simulink model "TestaBlocosUteis2"  (R2020b)
settings: Solver=FixedStepDiscrete  StartTime=0.0  StopTime=Plano.Tempo(end)  FixedStep=1  RelTol=1e-3
InitFcn:
  | CarregaTabelas
  | Plano=readtable('PlanoExperimentos.xlsx');
  | FreqIni=Plano.Frequencia(1);
  | PChegadaIni=Plano.PMonAlvo(1);
  | PSucIni=Interpola(FreqIni,PChegadaIni,TabSimulador,8);
  | VazaoIni=Interpola(FreqIni,PChegadaIni,TabSimulador,3);
  | FreqAlvoIni=FreqIni+1;
  | PMonAlvoIni=PChegadaIni+1;
  | VazaoAlvoIni=Interpola(FreqAlvoIni,PMonAlvoIni*1.019716,TabSimulador,3);
values from neighbouring files (symbols this model uses):
  BTP = readtable('DoBTP.xlsx')    [CarregaTabelas.m]
  TabSimulador = LeConverteNomes('DoSimulador.xlsx')    [CarregaTabelas.m]
undefined symbols (not defined in the file or in its folder): Interpola
settings Model: Creator=leize  LastModifiedBy=leize

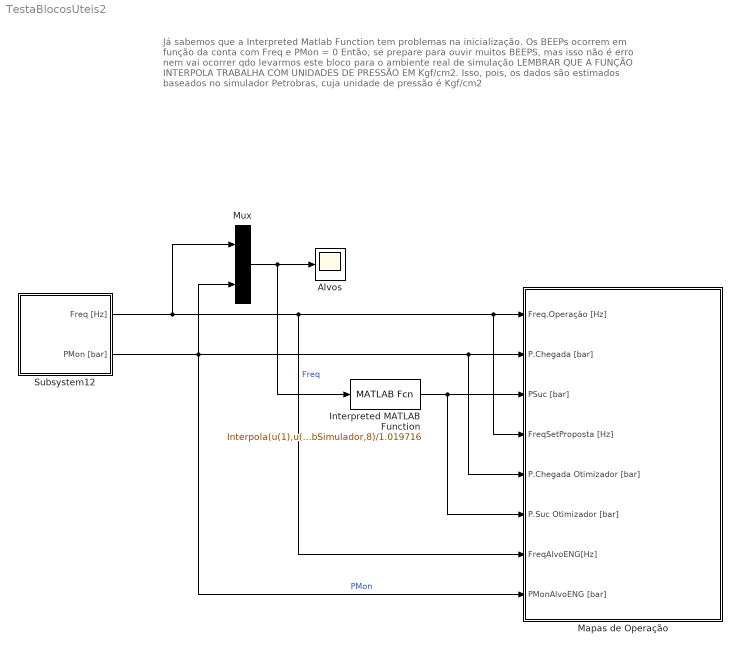
== system TestaBlocosUteis2 ==
  note: Já sabemos que a Interpreted Matlab Function tem problemas na inicialização.
      |
      | Os BEEPs ocorrem em função da conta com Freq e PMon = 0
      |
      | Então, se prepare para ouvir muitos BEEPS, mas isso não é erro nem vai ocorrer qdo levarmos este bloco para o ambiente real de simulação
      |
      | LEMBRAR QUE A FUNÇÃO INTERPOLA TRABALHA COM UNIDADES DE PRESSÃO EM Kgf/cm2. Isso, pois, os dados são estimados baseados no simulador Petrobras, cuja unidade de pressão é Kgf/cm2
  Alvos : Scope
  Interpreted MATLAB Function : MATLABFcn  MATLABFcn=Interpola(u(1),u(2)*1.019716,TabSimulador,8)/1.019716
  Mapas de Operação : Subsystem  mask{PlotaMapas=1, HabilitaRastro=1, Tsim=TabSimulador, BTP=BTP, FreqIni=FreqIni, PChegadaIni=PChegadaIni, PSucIni=PSucIni, FreqAlvoIni=FreqAlvoIni, PMonAlvoIni=PMonAlvoIni}
      mask prompts: PlotaMapas "Plotar Mapas (1/0)?"; HabilitaRastro "Habilita Rastro do Plot (1/0)?"; Tsim "Tabela do Simulador"; BTP "Tabela BTP"; FreqIni "Frequencia Inicial [Hz]"; PChegadaIni "PChegada Inicial [bar]"; PSucIni "Pressao de Succao Inicial [bar]"; FreqAlvoIni "Frequencia ALVO Inicial [Hz]"; PMonAlvoIni "PChegada ALVO [bar]"
      mask DialogControl DescTextVar Prompt: MAPAS DE OPERAÇÃO
      mask DialogControl ParameterGroupVar Prompt: Tabelas Petrobras e configurações dos Mapas de Operação
      mask DialogControl ParameterGroupVar_copy Prompt: Dados do Processo
      mask DialogControl ParameterGroupVar_copy_copy_copy Prompt: Dados Engenharia (Alvos)
  Mux : Mux  Inputs=2
  Subsystem12 : Subsystem  mask{Plano=Plano}
      mask prompts: Plano "Plano de Execucao"
      mask DialogControl DescGroupVar Prompt: TABELA COM PLANO DE EXECUCAO
  wires:
  Mux/1 -> Alvos/1, Interpreted MATLAB Function/1
  Subsystem12/2(PMon [bar]) -> Mapas de Operação/8(PMonAlvoENG [bar]), Mux/2, Mapas de Operação/5(P.Chegada Otimizador [bar]), Mapas de Operação/2(P.Chegada [bar])  "PMon"
  Subsystem12/1(Freq [Hz]) -> Mux/1, Mapas de Operação/7(FreqAlvoENG[Hz]), Mapas de Operação/4(FreqSetProposta [Hz]), Mapas de Operação/1(Freq.Operação [Hz])  "Freq"
  Interpreted MATLAB Function/1 -> Mapas de Operação/3(PSuc [bar]), Mapas de Operação/6(P.Suc Otimizador [bar])

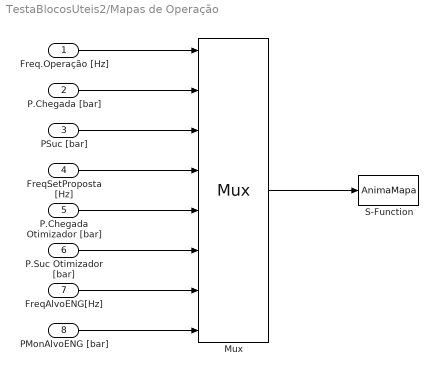
== system TestaBlocosUteis2/Mapas de Operação ==
  Freq.Operação [Hz] : Inport
  P.Chegada [bar] : Inport  Port=2
  PSuc [bar] : Inport  Port=3
  FreqSetProposta [Hz] : Inport  Port=4
  P.Chegada Otimizador [bar] : Inport  Port=5
  P.Suc Otimizador [bar] : Inport  Port=6
  FreqAlvoENG[Hz] : Inport  Port=7
  PMonAlvoENG [bar] : Inport  Port=8
  Mux : Mux  Inputs=8
  S-Function : S-Function  FunctionName=AnimaMapa  Parameters=PlotaMapas,Tsim,BTP,FreqIni, PChegadaIni,PSucIni,FreqAlvoIni,PMonAlvoIni,HabilitaRastro  SFunctionDeploymentMode=off  EnableBusSupport=off
  wires:
  Freq.Operação [Hz]/1 -> Mux/1
  Mux/1 -> S-Function/1
  P.Chegada [bar]/1 -> Mux/2
  PSuc [bar]/1 -> Mux/3
  P.Chegada Otimizador [bar]/1 -> Mux/5
  P.Suc Otimizador [bar]/1 -> Mux/6
  FreqAlvoENG[Hz]/1 -> Mux/7
  PMonAlvoENG [bar]/1 -> Mux/8
  FreqSetProposta [Hz]/1 -> Mux/4

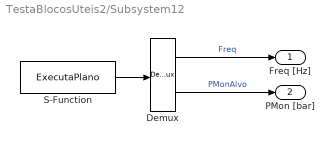
== system TestaBlocosUteis2/Subsystem12 ==
  Demux : Demux  Outputs=2
  S-Function : S-Function  FunctionName=ExecutaPlano  Parameters=Plano  SFunctionDeploymentMode=off  EnableBusSupport=off
  Freq [Hz] : Outport
  PMon [bar] : Outport  Port=2
  wires:
  S-Function/1 -> Demux/1
  Demux/1 -> Freq [Hz]/1  "Freq"
  Demux/2 -> PMon [bar]/1  "PMonAlvo"
